simulink subsystem "AUTOMATIC_ACK"  (R2022b)
settings: Solver=VariableStepAuto  StartTime=0.0  StopTime=10.0  RelTol=1e-3
settings Model: Creator=BEATOA  LastModifiedBy=BEATOA

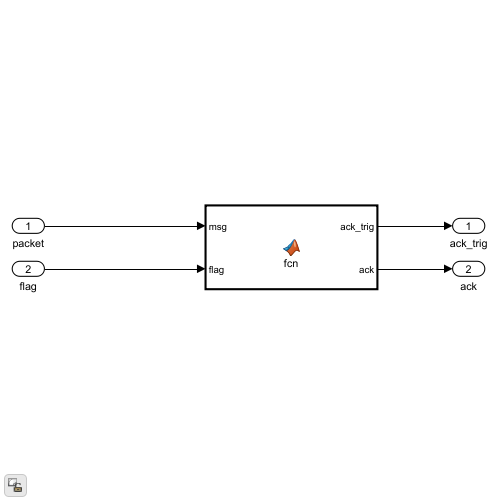
[thumbnail: Simulink's stored preview of the top-level diagram]
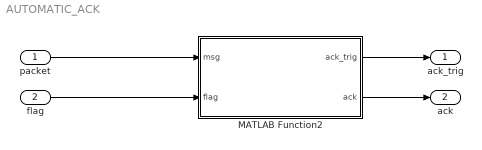
== system AUTOMATIC_ACK ==
  packet : Inport
  flag : Inport  Port=2
  MATLAB Function2 : MATLAB Function  TreatAsAtomicUnit=on
  ack_trig : Outport
  ack : Outport  Port=2
  wires:
  packet/1 -> MATLAB Function2/1(msg)
  MATLAB Function2/2(ack) -> ack/1
  MATLAB Function2/1(ack_trig) -> ack_trig/1
  flag/1 -> MATLAB Function2/2(flag)

== matlab function AUTOMATIC_ACK/MATLAB Function2 ==
  settings: updateMethod=DISCRETE
  data: ack_trig output; msg input uint8; ack output; flag input
function [ack_trig, ack]  = fcn(msg, flag)
% Message Decoding 
% WIN PACKET MESSAGE
% typedef struct
% {
% 1    uint8 dle;
% 2    uint8 stx;
% 
% 3    uint8 destination   :4;
% 3    uint8 source        :4;
% 
% 4    uint8 sap           :4;
% 4    uint8 msg_count     :4;
% 
% 5   uint8 sdu_length;
% 6   uint8 payload[WIN_MAX_OUTGOING_DATA_SIZE + 1]; // Data + CRC8
% } WIN_OUTGOING_MESSAGE_TYPE;
PAD_SIZE = 100;
% padding
packet_pad = zeros (PAD_SIZE,1);
ack = uint8(packet_pad);
ack_trig = 0;

if (flag)

    source      = bitshift(bitand(msg(3),hex2dec('0xF0')),-4);
    destination = bitand(msg(3),hex2dec('0x0F'));
    sap         = bitand(msg(4),hex2dec('0x0F'));
    sdu_length  = msg(5);
    
    reveal_msg = msg(6:6+sdu_length);
    
    % Reveal Message Decoding 
    %  1   uint8 api_id              ;                 //API number
    %  2   uint8 op_code           :5;                 //Opcode
    %  2   uint8 cmd_fb            :1;                 //Command/Feedback
    %  2   uint8 frag              :1;                 //Fragmentation
    %  2   uint8 mmp               :1;                 //More Message Pending
    %  3   uint8 payload[REVEAL_PAYLOAD_INCOMING_SIZE + REVEAL_LLC_CRC_SIZE];
    api         = reveal_msg(1);
    op_code     = bitand(reveal_msg(2), hex2dec('0x1F'));
    cmd_fb      = bitshift(bitand(reveal_msg(2), hex2dec('0x20')),-5);
    size        = sdu_length - 2;
    if (size >0)
        payload     = reveal_msg(3:3+size-1);
    else
        payload = [];
    end
        
    if (cmd_fb == 0)    
        % preparing ACK message
    
        % HEADER
        temp = destination;
        destination = source;
        source = temp;
        sdu_length = 5;   % Api 1- Opcode1 - ACK_response - API_ACK - OPCODE_ACK
        sap = 4;
        api_ack = api;
        op_code_ack = op_code;
        api_id = 1;
        op_code = 1;
        cmd_fb = 1;
        frag = 0;
        mmp = 0;
        destination_source = destination + source * (2^4);
        opcode_compl = op_code + cmd_fb * (2^5) + frag * (2^6) + mmp * (2^7);
    
        header_ack = uint8([destination_source sap sdu_length api_id opcode_compl]);
    
        ack_response = 0;
        crc_dummy = 0;
        packet_ack = uint8([header_ack ack_response api_ack op_code_ack crc_dummy]);
    
        ack(1:length(packet_ack)) = packet_ack;
        
        ack_trig = 1;
    end
end
